simulink model "fxpdemo_fpa"  (Simulink 7.6)
settings: Solver=ode4  SolverMode=SingleTasking  StartTime=0.0  StopTime=5  FixedStep=0.01  RelTol=1e-3  AbsTol=1e-6
Description:
  | Fixed-Point Advisor
  | 
  | This model highlights key features of the Fixed-Point Advisor (FPA), which complements the Fixed-Point
  | Tool (FPT).  The FPA facilitates converting a floating-point model or subsystem to an equivalent fixed-point
  | representation.  You can use the FPA to prepare a model for conversion and obtain an initial
  | scaling to use as the starting point for refinement and exploration inside the FPT.
settings Model: Perimeter=fxpdemo_feedback_STOOL/Controller_System/ControllerAlg  FileExcelVar=DD_Variable  FileExcelCalib=DD_Calib  vCheckAllBoolean=1  vCheckSumBase=1  vCheckProdBase=1  isChart=0  vCheckDoublesim=1  ASAP=1  vCheckPrecision=1  vSaveConf=1  InitialBaseType=7  InitialScaling=2^(-6)  Creator=The MathWorks Inc.  CovMetricSettings=d  ExtModeTrigMode=oneshot  ExtModeArmWhenConnect=off  ExtModeAutoUpdateStatusClock=off
settings SolverCC: InsertRTBMode=Auto
settings DataIOCC: LimitDataPoints=off  SignalLoggingName=sigsOut
settings OptimizationCC: BlockReduction=off  InlineParams=on  InlineInvariantSignals=on  InitFltsAndDblsToZero=on
settings DebuggingCC: SaveWithParameterizedLinksMsg=none  SolverPrmCheckMsg=none  MultiTaskDSMMsg=warning  MultiTaskCondExecSysMsg=none  IntegerOverflowMsg=none  ParameterDowncastMsg=warning  ParameterOverflowMsg=warning  ParameterPrecisionLossMsg=none  StrictBusMsg=ErrorOnBusTreatedAsVector
settings HardwareCC: ProdHWDeviceType=Generic->Unspecified (assume 32-bit Generic)
settings SFSimCC: SimParseCustomCode=off
settings RTWCC: GenerateReport=on  RTWVerbose=off  IncludeERTFirstTime=on
settings CodeAppCC: GenerateComments=off  IncDataTypeInIds=on  SimulinkBlockComments=off
settings GRTTargetCC: TargetFcnLib=ansi_tfl_tmw.mat

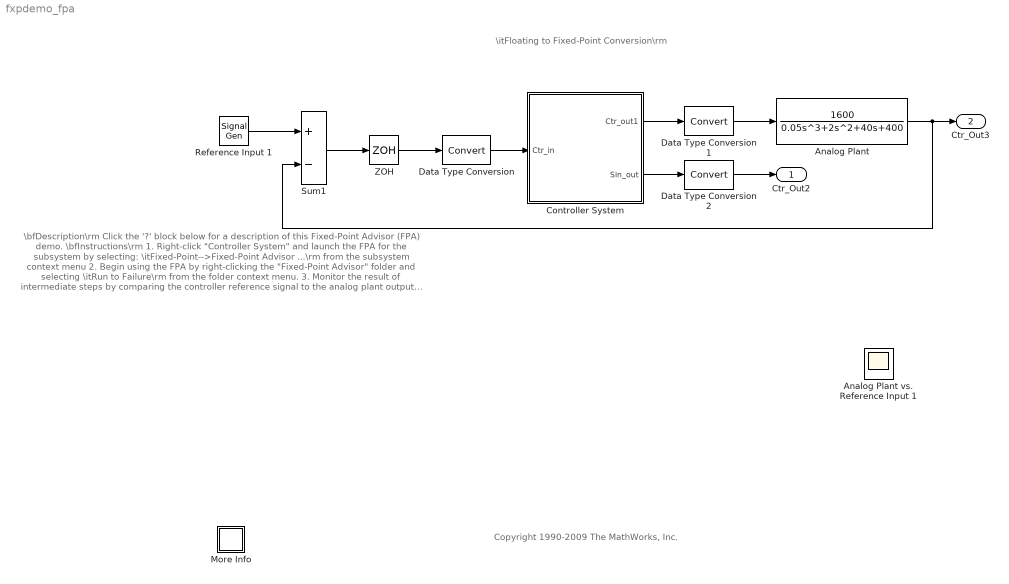
== system fxpdemo_fpa ==
  note: \bfDescription\rm
      | Click the '?' block below for a description of this Fixed-Point Advisor (FPA) demo.
      |
      | \bfInstructions\rm
      | 1. Right-click "Controller System" and launch the FPA for the subsystem by selecting:
      |     \itFixed-Point-->Fixed-Point Advisor ...\rm from the subsystem context menu
      | 2. Begin using the FPA by right-clicking the "Fixed-Point Advisor" folder and selecting
      |     \itRun to Failure\rm from the folder context menu.
      | 3. Monitor the result of intermediate steps by comparing the controller reference signal
      |     to the analog plant output signal using the floating scope to the right.
      |
      | \bfHint\rm
      | 1. When prompted, set output minimum and maximum values for inport Ctr\_in to -5 and 5,
      |     respectively.
      | 2. Data Type Conversion blocks have been placed around "Controller System" to
      |     decouple data type requirements between the plant and the controller.
  note: Copyright 1990-2009 The MathWorks, Inc.
  note: \itFloating to Fixed-Point Conversion\rm
  Analog Plant : TransferFcn  Numerator=1600  Denominator=[0.05, 2, 40, 400]
  Analog Plant vs. Reference Input 1 : Scope
      settings: Floating=on  TickLabels=on  TimeRange=5
  Controller System : Subsystem
      settings: RTWMemSecFuncInitTerm=Default  RTWMemSecFuncExecute=Default  RTWMemSecDataConstants=Default  RTWMemSecDataInternal=Default  RTWMemSecDataParameters=Default
  Data Type Conversion : DataTypeConversion
  Data Type Conversion1 : DataTypeConversion
  Data Type Conversion2 : DataTypeConversion
  More Info : Subsystem
      settings: OpenFcn=showdemo(bdroot(gcs))
      mask Display: disp('?')
  Reference Input 1 : SignalGenerator  WaveForm=square  Amplitude=2  Frequency=0.25
  Sum1 : Sum  Inputs=+-  SaturateOnIntegerOverflow=on  InputSameDT=on  OutDataTypeStr=Inherit: Same as first input
  ZOH : ZeroOrderHold  SampleTime=0.01
  Ctr_Out2 : Outport
  Ctr_Out3 : Outport  Port=2
  wires:
  Reference Input 1/1 -> Sum1/1
  Analog Plant/1 -> Sum1/2, Ctr_Out3/1
  Sum1/1 -> ZOH/1
  Controller System/1(Ctr_out1) -> Data Type Conversion1/1
  ZOH/1 -> Data Type Conversion/1
  Controller System/2(Sin_out) -> Data Type Conversion2/1
  Data Type Conversion/1 -> Controller System/1(Ctr_in)
  Data Type Conversion1/1 -> Analog Plant/1
  Data Type Conversion2/1 -> Ctr_Out2/1

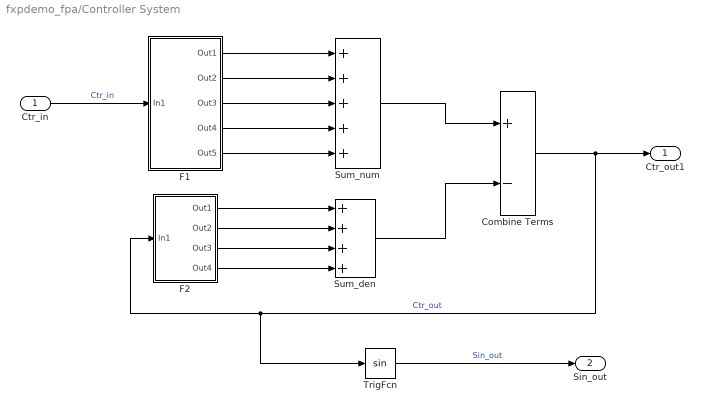
== system fxpdemo_fpa/Controller System ==
  Ctr_in : Inport
  Combine Terms : Sum  Inputs=+-  SaturateOnIntegerOverflow=on
  F1 : Subsystem
  F2 : Subsystem
  Sum_den : Sum  Inputs=++++  SaturateOnIntegerOverflow=on
  Sum_num : Sum  Inputs=+++++  SaturateOnIntegerOverflow=on
  TrigFcn : Trigonometry
  Ctr_out1 : Outport
  Sin_out : Outport  Port=2
  wires:
  F2/4(Out4) -> Sum_den/4
  F2/3(Out3) -> Sum_den/3
  F2/2(Out2) -> Sum_den/2
  F2/1(Out1) -> Sum_den/1
  Sum_num/1 -> Combine Terms/1
  Sum_den/1 -> Combine Terms/2
  Combine Terms/1 -> Ctr_out1/1, F2/1(In1), TrigFcn/1  "Ctr_out"
  TrigFcn/1 -> Sin_out/1  "Sin_out"
  Ctr_in/1 -> F1/1(In1)  "Ctr_in"
  F1/1(Out1) -> Sum_num/1
  F1/2(Out2) -> Sum_num/2
  F1/3(Out3) -> Sum_num/3
  F1/4(Out4) -> Sum_num/4
  F1/5(Out5) -> Sum_num/5

== system fxpdemo_fpa/More Info ==

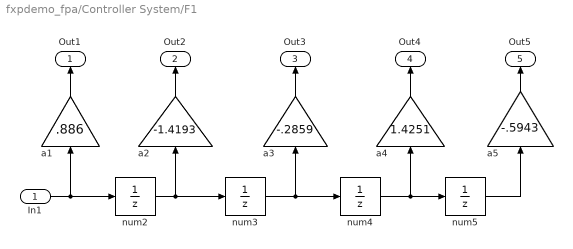
== system fxpdemo_fpa/Controller System/F1 ==
  In1 : Inport
  a1 : Gain  Gain=.886  SaturateOnIntegerOverflow=on  OutDataTypeStr=Inherit: Same as input
  a2 : Gain  Gain=-1.4193  SaturateOnIntegerOverflow=on  OutDataTypeStr=Inherit: Same as input
  a3 : Gain  Gain=-.2859  SaturateOnIntegerOverflow=on  OutDataTypeStr=Inherit: Same as input
  a4 : Gain  Gain=1.4251  SaturateOnIntegerOverflow=on  OutDataTypeStr=Inherit: Same as input
  a5 : Gain  Gain=-.5943  SaturateOnIntegerOverflow=on  OutDataTypeStr=Inherit: Same as input
  num{2..5} (4 alike) : UnitDelay  X0=0.0  SampleTime=0.01
  Out1 : Outport
  Out2 : Outport  Port=2
  Out3 : Outport  Port=3
  Out4 : Outport  Port=4
  Out5 : Outport  Port=5
  wires:
  num5/1 -> a5/1
  num4/1 -> a4/1, num5/1
  num3/1 -> a3/1, num4/1
  num2/1 -> a2/1, num3/1
  In1/1 -> num2/1, a1/1
  a4/1 -> Out4/1
  a1/1 -> Out1/1
  a3/1 -> Out3/1
  a2/1 -> Out2/1
  a5/1 -> Out5/1

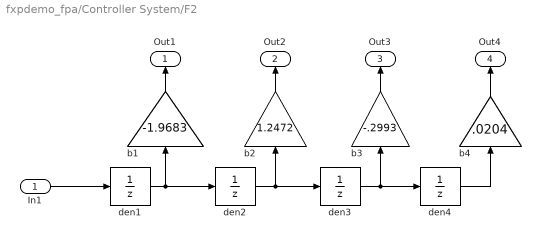
== system fxpdemo_fpa/Controller System/F2 ==
  In1 : Inport
  b1 : Gain  Gain=-1.9683  SaturateOnIntegerOverflow=on  OutDataTypeStr=Inherit: Same as input
  b2 : Gain  Gain=1.2472  SaturateOnIntegerOverflow=on  OutDataTypeStr=Inherit: Same as input
  b3 : Gain  Gain=-.2993  SaturateOnIntegerOverflow=on  OutDataTypeStr=Inherit: Same as input
  b4 : Gain  Gain=.0204  SaturateOnIntegerOverflow=on  OutDataTypeStr=Inherit: Same as input
  den{1..4} (4 alike) : UnitDelay  X0=0.0  SampleTime=0.01
  Out1 : Outport
  Out2 : Outport  Port=2
  Out3 : Outport  Port=3
  Out4 : Outport  Port=4
  wires:
  den1/1 -> b1/1, den2/1
  den4/1 -> b4/1
  den3/1 -> b3/1, den4/1
  den2/1 -> b2/1, den3/1
  In1/1 -> den1/1
  b1/1 -> Out1/1
  b2/1 -> Out2/1
  b3/1 -> Out3/1
  b4/1 -> Out4/1
